simulink model "mppt1"  (R2024a)
settings: Solver=ode23tb  StartTime=0.0  StopTime=3  RelTol=1e-3
undefined symbols (not defined in the file): Acid, Lead
libraries: spsSeriesRLCBranchLib x3, spsBatteryLib x1, spsDiodeLib x1, spsGroundLib x1, spsMosfetLib x1, spsPVArrayLib x1, spsPWMGeneratorDCDCLib x1, sps_lib x1
settings Model: Creator=hp  LastModifiedBy=hp

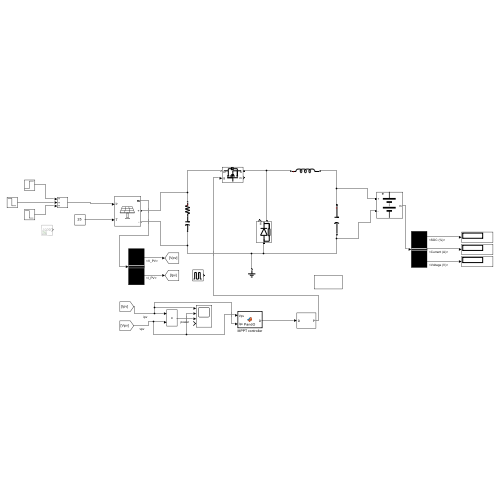
[thumbnail: Simulink's stored preview of the top-level diagram]
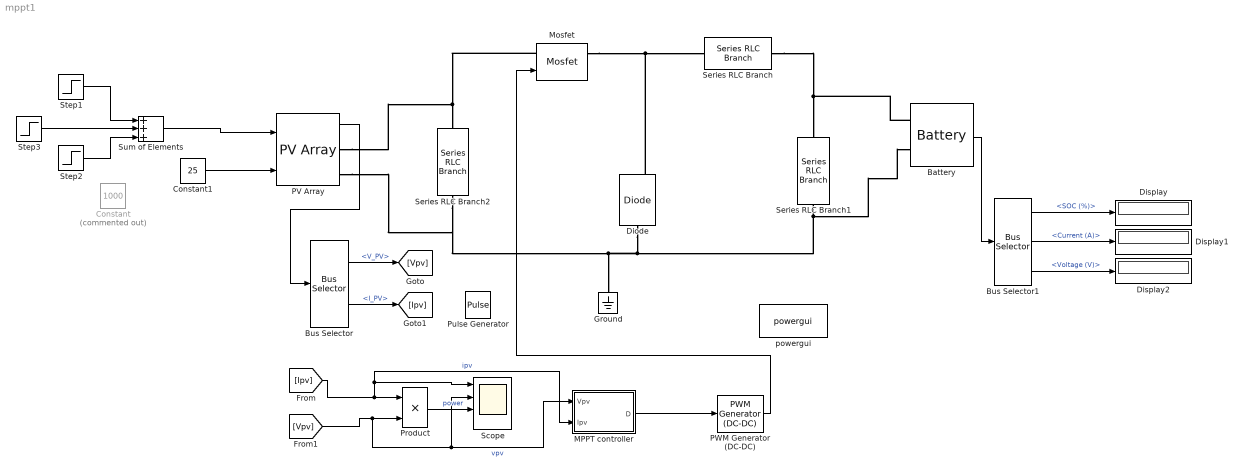
== system mppt1 ==
  Battery : spsBatteryLib/Battery  BatType=Lead-Acid  ShowTempParam=off  ThermalPreset=no  ShowAgeParam=off  NomV=12  NomQ=7  SOC=41  Batt_Tr=30  PresetModel=on  MaxQ=7.2917  MinV=9  FullV=13.0658  Dis_rate=1.4  R=0.017143  Normal_OP=2.1719  expZone="[12.2171    0.0233333]"  current=[6.5 13 32.5]  Units=Time  Tci=20  NomT=20  T2=-30  MaxQ2=4.8  FullV2=7.1  Normal_OP2=5.655  expZone2="[6.58           1]"  Rca=0.6  ti=2000  Dp=0  Neq0=0  Tsim=1e6  Ta1=25  Qeol=5.4*0.9  Reol=0.013333*1.2  Char_age=[2.3478, 3]  Dis_age=[2.3478, 10]  N1=1500  N2=10500  N3=1000  N4=1400  Ta2=45  N5=950
  Bus Selector : BusSelector  OutputSignals=V_PV,I_PV
  Bus Selector1 : BusSelector  OutputSignals=SOC (%),Current (A),Voltage (V)
  Constant : Constant  Commented=on  Value=1000
  Constant1 : Constant  Value=25
  Diode : spsDiodeLib/Diode  Ron=0.001  Lon=0  Vf=0.8  IC=0  UseSnubber=0  Rs=500  Cs=250e-9  Measurements=on
  Display : Display
  Display1 : Display
  Display2 : Display
  Ground : spsGroundLib/Ground  LConnTagsString=a
  MPPT controller : MATLAB Function  TreatAsAtomicUnit=on
  Mosfet : spsMosfetLib/Mosfet  Ron=0.1  Lon=0  Rd=0.01  Vfd=0  IC=0  Rs=1e5  Cs=inf  Measurements=on
  PV Array : spsPVArrayLib/PV Array  Npar=1  Nser=1  PlotType=one module @ 25 deg.C & specified irradiances  S_vec="[ 1000  500  100 ]"  Temp_C_vec="[ 45 25  ]"  ModuleName=User-defined  PlotWhenSelected=off  Pm=50.04  Ncell=36  Voc=22  Isc=3  Vm=18  Im=2.78  beta_Voc_pc=-0.36099  alpha_Isc_pc=0.102  beta_Voc=-0.079418  alpha_Isc=0.00306  IL=3.0055  I0=1.1133e-10  nI=0.99152  Rsh=251.1908  Rs=0.45699  RobustModel=off  RobustCellTemperature=313.3991  BAL=on  Tc=1e-6  Tfilter=5e-5
  PWM Generator (DC-DC) : spsPWMGeneratorDCDCLib/PWM Generator (DC-DC)  Fsw=100000  Ts=1e-6
  Product : Product
  Pulse Generator : DiscretePulseGenerator  PulseType=Time based  Period=10e-6  PulseWidth=78
  Scope : Scope  NumInputPorts=4
  Series RLC Branch : spsSeriesRLCBranchLib/Series RLC Branch  LConnTagsString=__new0  RConnTagsString=__new0  BranchType=L  Resistance=1  Inductance=100e-6  SetiL0=off  InitialCurrent=0  Capacitance=1e-6  Setx0=off  InitialVoltage=0  Measurements=None
  Series RLC Branch1 : spsSeriesRLCBranchLib/Series RLC Branch  LConnTagsString=__new0  RConnTagsString=__new0  BranchType=C  Resistance=1  Inductance=1e-3  SetiL0=off  InitialCurrent=0  Capacitance=470e-6  Setx0=off  InitialVoltage=0  Measurements=None
  Series RLC Branch2 : spsSeriesRLCBranchLib/Series RLC Branch  LConnTagsString=__new0  RConnTagsString=__new0  BranchType=RC  Resistance=0.001  Inductance=1e-3  SetiL0=off  InitialCurrent=0  Capacitance=1000e-6  Setx0=off  InitialVoltage=0  Measurements=None
  Step1 : Step  Time=0  After=1000  SampleTime=0
  Step2 : Step  Time=2  After=-200  SampleTime=0
  Step3 : Step  After=-200  SampleTime=0
  Sum of Elements : Sum  Inputs=+++
  powergui : sps_lib/powergui  Priority=1  SimulationMode=Discrete  SampleTime=1e-6  frequency=60  Iterations=50  frequencyindice=0  Pbase=100e6  ErrMax=1e-4  UnitsV=kV  UnitsW=MW  buscounter=0  FunctionMessages=off  echomessages=off  EnableUseOfTLC=off  CurrentSourceSwitches=off  DisableSnubberDevices=off  DisableRonSwitches=off  DisableVfSwitches=off  DisplayEquations=off  AutomaticDiscreteSolvers=off  SolverType=Tustin/Backward Euler (TBE)  Interpol=off  ExternalGateDelay=off  methode=off  Ts=100  x0status=blocks  SPID=on  SwTol=0  HookPort=off  NonlinearTolerance=1e-4  nMaxIteration=100  ContinueOnMaxIteration=off  RestoreLinks=warning  ResistiveCurrentMeasurement=off  Frange=[0:2:500]  Ylog=off  Xlog=on  ShowGrid=off  save=off  variable=ZData  structure=0  ZoomFFT=off  StartTime=0.0  cycles=1  DisplayStyle=1  fundamental=60  FreqAxis=off  MaxFrequency=1000  frequencyindicesteady=1  RmsSteady=1  display=off
  wires:
  Constant1/1 -> PV Array/2
  PV Array/1 -> Bus Selector/1
  Bus Selector/1 -> [Vpv]  "<V_PV>"
  Bus Selector/2 -> [Ipv]  "<I_PV>"
  [Ipv] -> Product/1, Scope/1, MPPT controller/2(Ipv)  "ipv"
  [Vpv] -> Product/2, Scope/2, MPPT controller/1(Vpv)  "vpv"
  Product/1 -> Scope/3  "power"
  Battery/1 -> Bus Selector1/1
  Bus Selector1/1 -> Display/1  "<SOC (%)>"
  Bus Selector1/3 -> Display2/1  "<Voltage (V)>"
  Bus Selector1/2 -> Display1/1  "<Current (A)>"
  Sum of Elements/1 -> PV Array/1
  MPPT controller/1(D) -> PWM Generator (DC-DC)/1
  PWM Generator (DC-DC)/1 -> Mosfet/1
  Step3/1 -> Sum of Elements/2
  Step2/1 -> Sum of Elements/3
  Step1/1 -> Sum of Elements/1
  connections:
  Mosfet/LConn1 -- PV Array/RConn1 -- Series RLC Branch2/LConn1
  Diode/LConn1 -- Ground/LConn1 -- PV Array/RConn2 -- Series RLC Branch2/RConn1 -- Battery/LConn2 -- Series RLC Branch1/RConn1
  Mosfet/RConn1 -- Diode/RConn1 -- Series RLC Branch/LConn1
  Series RLC Branch/RConn1 -- Battery/LConn1 -- Series RLC Branch1/LConn1

== matlab function mppt1/MPPT controller ==
  data: Vpv input; Ipv input; D output
function D = PandO(Vpv,Ipv)

persistent Dprev Pprev Vprev

if isempty(Dprev)
    Dprev = 0.5;
    Vprev = 18;
    Pprev = 50;
end

% Calculate power
Ppv = Vpv * Ipv;

% P&O Algorithm
if (Ppv - Pprev) ~= 0
    
    if (Ppv - Pprev) > 0
        
        if (Vpv - Vprev) > 0
            D = Dprev - 0.00005;
        else
            D = Dprev + 0.00005;
        end
        
    else
        
        if (Vpv - Vprev) > 0
            D = Dprev + 0.00005;
        else
            D = Dprev - 0.00005;
        end
        
    end
    
else
    D = Dprev;
end


% Limit duty between 0.1 and 0.9
if D > 0.85
    D = 0.78;
end

if D < 0.2
    D = 0.2;
end


% Update values
Dprev = D;
Vprev = Vpv;
Pprev = Ppv;
